simulink model "pointing"  (R2020b)
settings: Solver=ode15s  StartTime=9000  StopTime=15000  MaxStep=1  RelTol=1e-8  AbsTol=1e-8
values from neighbouring files (symbols this model uses):
  data = struct()    [config.m]    (also in config6U.m; configSlew.m; mainOffNominal.m = dataFix; statisticalAnalysis.m = dataFix)
settings Model: SimulationMode=accelerator  Creator=pacif  LastModifiedBy=pacif

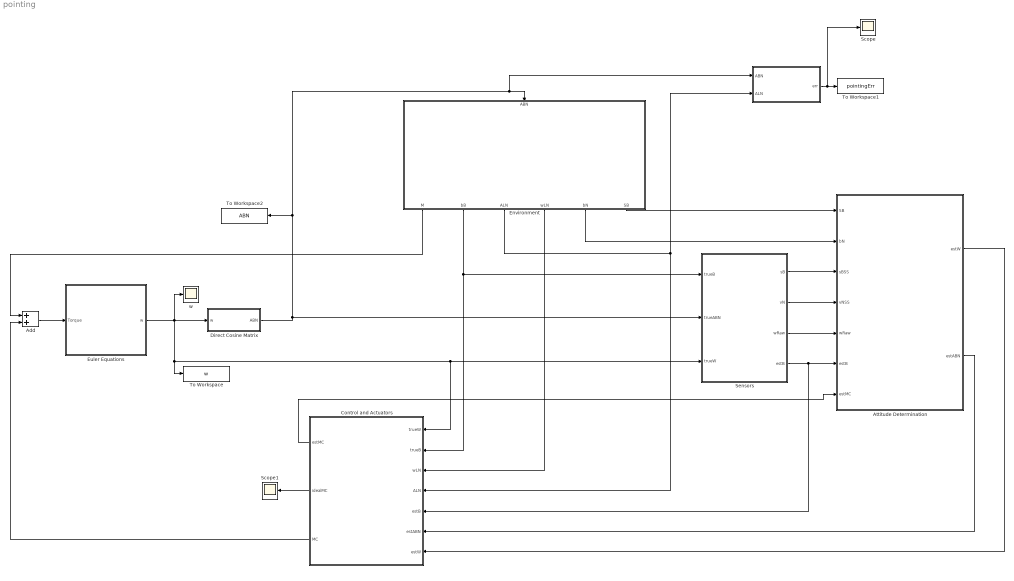
== system pointing ==
  " " : MATLAB Function  TreatAsAtomicUnit=on
  Add : Sum
  Attitude Determination : Subsystem
  Control and Actuators : Subsystem  AncestorBlock=libraryMatlab/Control Logic
  Direct Cosine Matrix : Subsystem  AncestorBlock=libraryMatlab/Direct Cosine Matrix
  Environment : Subsystem  AncestorBlock=libraryMatlab/Environment
  Euler Equations : Subsystem  AncestorBlock=libraryMatlab/Euler Equations
  Scope : Scope
  Scope1 : Scope
  Sensors : Subsystem  AncestorBlock=libraryMatlab/Sensors Old
  To Workspace : ToWorkspace  VariableName=w  SaveFormat=Timeseries  SampleTime=-1
  To Workspace1 : ToWorkspace  VariableName=pointingErr  SaveFormat=Timeseries  SampleTime=-1
  To Workspace2 : ToWorkspace  VariableName=ABN  SaveFormat=Timeseries  SampleTime=-1
  w : Scope
  wires:
  Environment/2(bB) -> Sensors/1(trueB), Control and Actuators/2(trueB)
  Add/1 -> Euler Equations/1(Torque)
  Environment/1(M) -> Add/1
  Euler Equations/1(w) -> Direct Cosine Matrix/1(w), To Workspace/1, Sensors/3(trueW), Control and Actuators/1(trueW), w/1
  Direct Cosine Matrix/1(ABN) -> Sensors/2(trueABN), To Workspace2/1, Environment/1(ABN), " "/1(ABN)
  Environment/3(ALN) -> " "/2(ALN), Control and Actuators/4(ALN)
  Environment/4(wLN) -> Control and Actuators/3(wLN)
  Control and Actuators/3(MC) -> Add/2
  Sensors/1(sB) -> Attitude Determination/3(sBSS)
  Sensors/2(vN) -> Attitude Determination/4(vNSS)
  Sensors/3(wRaw) -> Attitude Determination/5(wRaw)
  Sensors/4(estB) -> Control and Actuators/5(estB), Attitude Determination/6(estB)
  Control and Actuators/1(estMC) -> Attitude Determination/7(estMC)
  Environment/6(SB) -> Attitude Determination/1(SB)
  Environment/5(bN) -> Attitude Determination/2(bN)
  " "/1(err) -> Scope/1, To Workspace1/1
  Attitude Determination/2(estABN) -> Control and Actuators/6(estABN)
  Attitude Determination/1(estW) -> Control and Actuators/7(estW)
  Control and Actuators/2(idealMC) -> Scope1/1

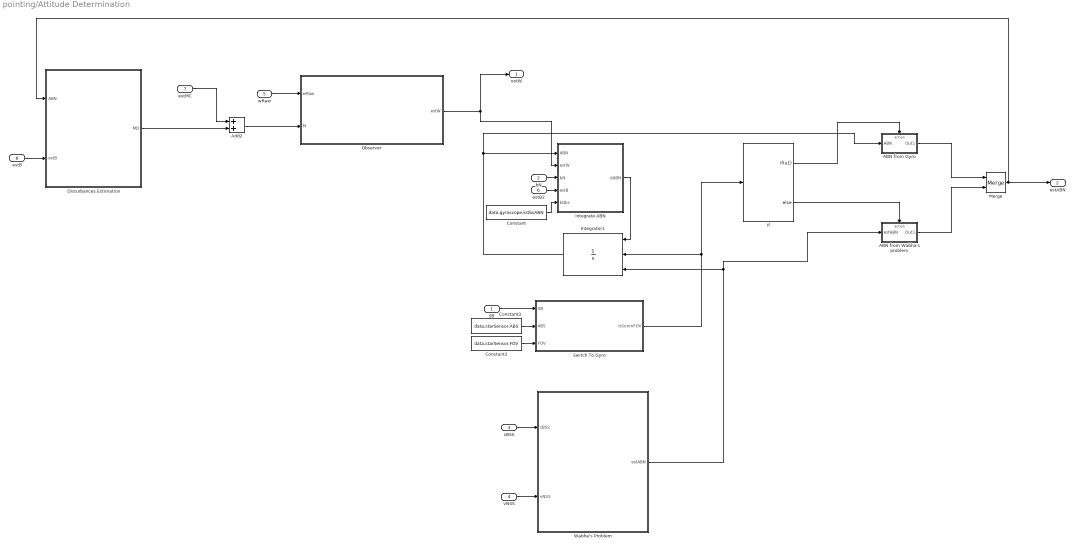
== system pointing/Attitude Determination ==
  SB : Inport
  bN : Inport  Port=2
  sBSS : Inport  Port=3
  vNSS : Inport  Port=4
  wRaw : Inport  Port=5
  estB : Inport  Port=6
  estMC : Inport  Port=7
  ABN from Gyro : Subsystem  TreatAsAtomicUnit=on
  ABN from Wabha's problem : Subsystem  TreatAsAtomicUnit=on
  Add2 : Sum
  Constant : Constant  Value=data.gyroscope.kObsABN
  Constant2 : Constant  Value=data.starSensor.FOV
  Constant3 : Constant  Value=data.starSensor.ABS
  Disturbances Estimation : Subsystem  AncestorBlock=libraryMatlab/Environment
  If : If  IfExpression=u1
  Integrate ABN : MATLAB Function  TreatAsAtomicUnit=on
  Integrator1 : Integrator  ExternalReset=either  InitialConditionSource=external
  Merge : Merge
  Observer : Subsystem
  Switch To Gyro : MATLAB Function  AncestorBlock=libraryMatlab/Is Sun in FOV?  TreatAsAtomicUnit=on
  Wabha's Problem : MATLAB Function  TreatAsAtomicUnit=on
  estB2 : InportShadow  Port=6
  estW : Outport
  estABN : Outport  Port=2
  wires:
  estB/1 -> Disturbances Estimation/2(estB)
  Observer/1(estW) -> estW/1, Integrate ABN/2(estW)
  Add2/1 -> Observer/2(M)
  Disturbances Estimation/1(MD) -> Add2/2
  wRaw/1 -> Observer/1(wRaw)
  estMC/1 -> Add2/1
  Switch To Gyro/1(isSunInFOV) -> If/1, Integrator1/2
  SB/1 -> Switch To Gyro/1(SB)
  Constant2/1 -> Switch To Gyro/3(FOV)
  Constant3/1 -> Switch To Gyro/2(ABS)
  ABN from Wabha's problem/1(Out1) -> Merge/2
  sBSS/1 -> Wabha's Problem/1(sBSS)
  Merge/1 -> Disturbances Estimation/1(ABN), estABN/1
  If/1 -> ABN from Gyro/Action
  Integrator1/1 -> Integrate ABN/1(ABN), ABN from Gyro/1(ABN)
  If/2 -> ABN from Wabha's problem/Action
  Integrate ABN/1(dABN) -> Integrator1/1
  vNSS/1 -> Wabha's Problem/2(vNSS)
  ABN from Gyro/1(Out1) -> Merge/1
  Wabha's Problem/1(estABN) -> ABN from Wabha's problem/1(estABN), Integrator1/3
  bN/1 -> Integrate ABN/3(bN)
  estB2/1 -> Integrate ABN/4(estB)
  Constant/1 -> Integrate ABN/5(kObs)

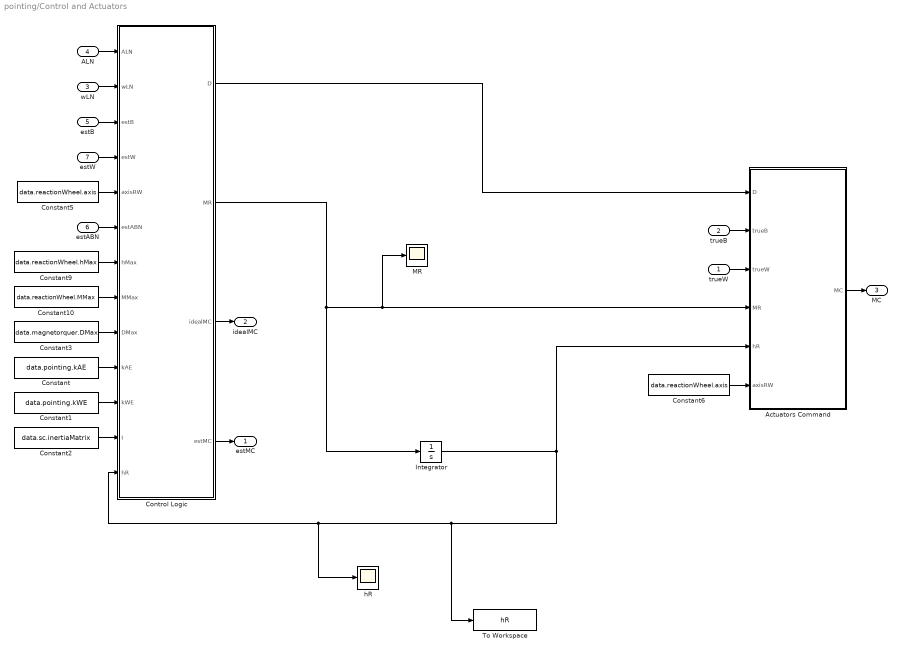
== system pointing/Control and Actuators ==
  trueW : Inport
  trueB : Inport  Port=2
  wLN : Inport  Port=3
  ALN : Inport  Port=4
  estB : Inport  Port=5
  estABN : Inport  Port=6
  estW : Inport  Port=7
  Actuators Command : MATLAB Function  TreatAsAtomicUnit=on
  Constant : Constant  Value=data.pointing.kAE
  Constant1 : Constant  Value=data.pointing.kWE
  Constant10 : Constant  Value=data.reactionWheel.MMax
  Constant2 : Constant  Value=data.sc.inertiaMatrix
  Constant3 : Constant  Value=data.magnetorquer.DMax
  Constant5 : Constant  Value=data.reactionWheel.axis
  Constant6 : Constant  Value=data.reactionWheel.axis
  Constant9 : Constant  Value=data.reactionWheel.hMax
  Control Logic : MATLAB Function  TreatAsAtomicUnit=on
  Integrator : Integrator  InitialCondition=data.reactionWheel.h0
  MR : Scope
  To Workspace : ToWorkspace  VariableName=hR  SaveFormat=Timeseries  SampleTime=-1
  hR : Scope
  estMC : Outport
  idealMC : Outport  Port=2  PortDimensions=3
  MC : Outport  Port=3
  wires:
  estB/1 -> Control Logic/3(estB)
  Constant2/1 -> Control Logic/12(I)
  wLN/1 -> Control Logic/2(wLN)
  estABN/1 -> Control Logic/6(estABN)
  estW/1 -> Control Logic/4(estW)
  Control Logic/3(idealMC) -> idealMC/1
  ALN/1 -> Control Logic/1(ALN)
  Constant5/1 -> Control Logic/5(axisRW)
  Constant3/1 -> Control Logic/9(DMax)
  Actuators Command/1(MC) -> MC/1
  trueB/1 -> Actuators Command/2(trueB)
  Constant6/1 -> Actuators Command/6(axisRW)
  trueW/1 -> Actuators Command/3(trueW)
  Constant9/1 -> Control Logic/7(hMax)
  Constant10/1 -> Control Logic/8(MMax)
  Control Logic/4(estMC) -> estMC/1
  Control Logic/1(D) -> Actuators Command/1(D)
  Control Logic/2(MR) -> Integrator/1, MR/1, Actuators Command/4(MR)
  Integrator/1 -> To Workspace/1, hR/1, Control Logic/13(hR), Actuators Command/5(hR)
  Constant/1 -> Control Logic/10(kAE)
  Constant1/1 -> Control Logic/11(kWE)

== system pointing/Direct Cosine Matrix ==
  w : Inport
  Integrator : Integrator  InitialCondition=data.ic.dcm
  MATLAB Function : MATLAB Function  TreatAsAtomicUnit=on
  MATLAB Function1 : MATLAB Function  TreatAsAtomicUnit=on
  ABN : Outport
  wires:
  MATLAB Function1/1(A) -> MATLAB Function/1(A), ABN/1
  Integrator/1 -> MATLAB Function1/1(A0)
  MATLAB Function/1(dA) -> Integrator/1
  w/1 -> MATLAB Function/2(w)

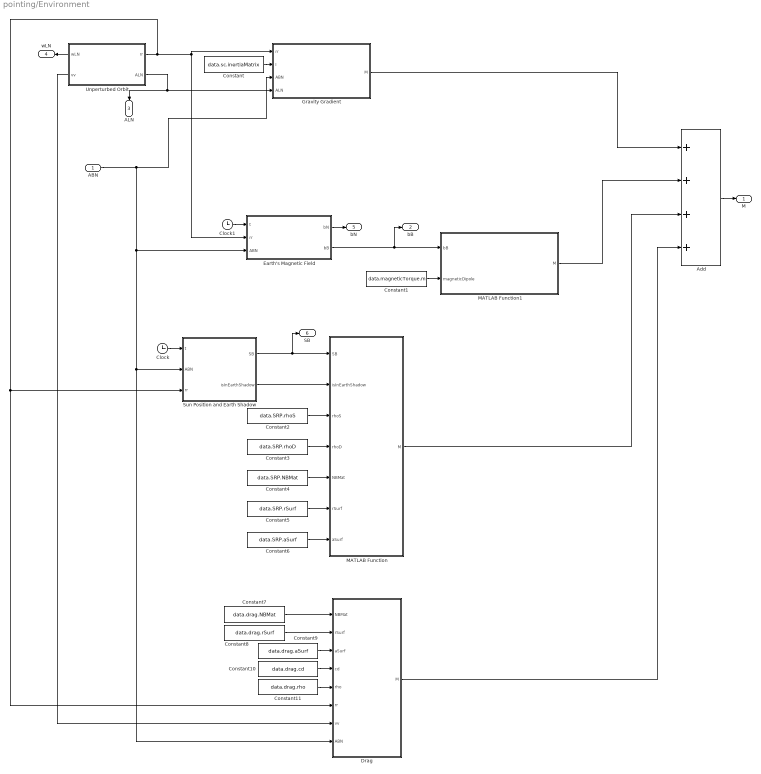
== system pointing/Environment ==
  ABN : Inport
  Add : Sum  Inputs=++++
  Clock : Clock
  Clock1 : Clock
  Constant : Constant  Value=data.sc.inertiaMatrix
  Constant1 : Constant  Value=data.magneticTorque.m
  Constant10 : Constant  Value=data.drag.cd
  Constant11 : Constant  Value=data.drag.rho
  Constant2 : Constant  Value=data.SRP.rhoS
  Constant3 : Constant  Value=data.SRP.rhoD
  Constant4 : Constant  Value=data.SRP.NBMat
  Constant5 : Constant  Value=data.SRP.rSurf
  Constant6 : Constant  Value=data.SRP.aSurf
  Constant7 : Constant  Value=data.drag.NBMat
  Constant8 : Constant  Value=data.drag.rSurf
  Constant9 : Constant  Value=data.drag.aSurf
  Drag : MATLAB Function  TreatAsAtomicUnit=on
  Earth's Magnetic Field : MATLAB Function  TreatAsAtomicUnit=on
  Gravity Gradient : MATLAB Function  TreatAsAtomicUnit=on
  MATLAB Function : MATLAB Function  TreatAsAtomicUnit=on
  MATLAB Function1 : MATLAB Function  TreatAsAtomicUnit=on
  Sun Position and Earth Shadow : MATLAB Function  TreatAsAtomicUnit=on
  Unperturbed Orbit : Subsystem
      settings: PortSchema="{\"entries\":[{\"content\":{\"sides\":[{\"content\":{\"connectorIds\":[\"Out3\",\"Out4\"]},\"type\":\"ConnectorPlacement.EquallySpacedRectSide\",\"uuid\":\"7ed69275-e977-4f2a-8fd3-997b16b83aea\"},{\"content\":{\"connectorIds\":[\"Out1\",\"Out2\"],\"side\":\"RIGHT\"},\"type\":\"ConnectorPlacement.EquallySpacedRectSide\",\"uuid\":\"1b6f9d42-4fef-4598-ba05-7b049053efd9\"},{\"content\":{\"connectorIds\":[],\"side\":\"TOP\"},\"type\":\"ConnectorPlacement.EquallySpacedRectSide\",\"uuid\":\"4e0c3aba-8d31-4992-bec6-35e5e83e5744\"},{\"content\":{\"connectorIds\":[],\"side\":\"HIDDEN\"},\"type\":\"ConnectorPlacement.EquallySpacedRectSide\",\"uuid\":\"810122fe-3bdf-4514-9a6d-d70c18985587\"}]},\"type\":\"ConnectorPlacement.EquallySpacedConnector\",\"uuid\":\"14af5646-8a65-4661-98d5-d8bad349b4d9\"}],\"packageUris\":[\"http://schema.mathworks.com/mf0/Connector/R2020b\"],\"version\":\"1.0\"}"
  M : Outport
  bB : Outport  Port=2
  ALN : Outport  Port=3
  wLN : Outport  Port=4
  bN : Outport  Port=5
  SB : Outport  Port=6
  wires:
  Sun Position and Earth Shadow/1(SB) -> SB/1, MATLAB Function/1(SB)
  Clock/1 -> Sun Position and Earth Shadow/1(t)
  Constant4/1 -> MATLAB Function/5(NBMat)
  Constant6/1 -> MATLAB Function/7(aSurf)
  Constant3/1 -> MATLAB Function/4(rhoD)
  Constant2/1 -> MATLAB Function/3(rhoS)
  Constant5/1 -> MATLAB Function/6(rSurf)
  ABN/1 -> Drag/8(ABN), Sun Position and Earth Shadow/2(ABN), Earth's Magnetic Field/3(ABN), Gravity Gradient/3(ABN)
  Add/1 -> M/1
  MATLAB Function/1(M) -> Add/3
  Gravity Gradient/1(M) -> Add/1
  Earth's Magnetic Field/2(bB) -> MATLAB Function1/1(bB), bB/1
  MATLAB Function1/1(M) -> Add/2
  Constant1/1 -> MATLAB Function1/2(magneticDipole)
  Constant/1 -> Gravity Gradient/2(I)
  Unperturbed Orbit/2(ALN) -> Gravity Gradient/4(ALN), ALN/1
  Unperturbed Orbit/1(rr) -> Sun Position and Earth Shadow/3(rr), Drag/6(rr), Gravity Gradient/1(rr), Earth's Magnetic Field/2(rr)
  Unperturbed Orbit/3(wLN) -> wLN/1
  Clock1/1 -> Earth's Magnetic Field/1(t)
  Constant8/1 -> Drag/2(rSurf)
  Constant9/1 -> Drag/3(aSurf)
  Constant10/1 -> Drag/4(cd)
  Constant7/1 -> Drag/1(NBMat)
  Unperturbed Orbit/4(vv) -> Drag/7(vv)
  Earth's Magnetic Field/1(bN) -> bN/1
  Drag/1(M) -> Add/4
  Constant11/1 -> Drag/5(rho)
  Sun Position and Earth Shadow/2(isInEarthShadow) -> MATLAB Function/2(isInEarthShadow)

== system pointing/Euler Equations ==
  Torque : Inport
  Constant : Constant  Value=data.sc.inertiaMatrix
  Integrator : Integrator  InitialCondition=data.ic.w
  MATLAB Function : MATLAB Function  TreatAsAtomicUnit=on
  w : Outport
  wires:
  MATLAB Function/1(dw) -> Integrator/1
  Torque/1 -> MATLAB Function/2(M)
  Integrator/1 -> MATLAB Function/1(w), w/1
  Constant/1 -> MATLAB Function/3(I)

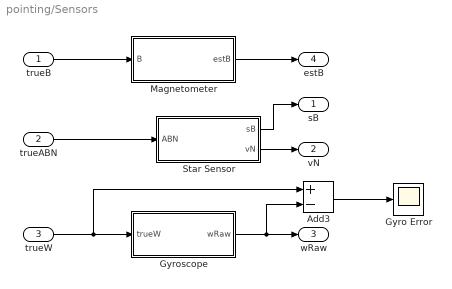
== system pointing/Sensors ==
  trueB : Inport
  trueABN : Inport  Port=2
  trueW : Inport  Port=3
  Add3 : Sum  Inputs=+-
  Gyro Error : Scope
  Gyroscope : Subsystem
  Magnetometer : Subsystem
  Star Sensor : Subsystem  AncestorBlock=libraryMatlab/Sensors/Star Sensor
  sB : Outport
  vN : Outport  Port=2
  wRaw : Outport  Port=3
  estB : Outport  Port=4
  wires:
  Magnetometer/1(estB) -> estB/1
  Add3/1 -> Gyro Error/1
  trueABN/1 -> Star Sensor/1(ABN)
  Star Sensor/1(sB) -> sB/1
  Star Sensor/2(vN) -> vN/1
  Gyroscope/1(wRaw) -> wRaw/1, Add3/2
  trueB/1 -> Magnetometer/1(B)
  trueW/1 -> Add3/1, Gyroscope/1(trueW)

== system pointing/Attitude Determination/ABN from Gyro ==
  ABN : Inport
  Action Port : ActionPort  ActionPortLabel=if(u1)
  Out1 : Outport
  wires:
  ABN/1 -> Out1/1

== system pointing/Attitude Determination/ABN from Wabha's problem ==
  estABN : Inport
  Action Port : ActionPort  ActionPortLabel=else
  Out1 : Outport
  wires:
  estABN/1 -> Out1/1

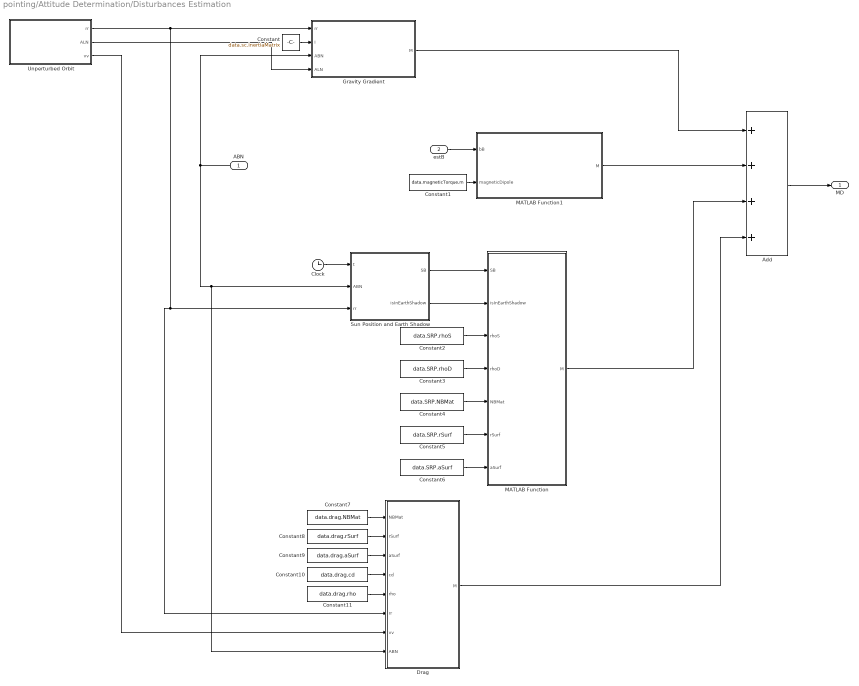
== system pointing/Attitude Determination/Disturbances Estimation ==
  ABN : Inport
  estB : Inport  Port=2
  Add : Sum  Inputs=++++
  Clock : Clock
  Constant : Constant  Value=data.sc.inertiaMatrix
  Constant1 : Constant  Value=data.magneticTorque.m
  Constant10 : Constant  Value=data.drag.cd
  Constant11 : Constant  Value=data.drag.rho
  Constant2 : Constant  Value=data.SRP.rhoS
  Constant3 : Constant  Value=data.SRP.rhoD
  Constant4 : Constant  Value=data.SRP.NBMat
  Constant5 : Constant  Value=data.SRP.rSurf
  Constant6 : Constant  Value=data.SRP.aSurf
  Constant7 : Constant  Value=data.drag.NBMat
  Constant8 : Constant  Value=data.drag.rSurf
  Constant9 : Constant  Value=data.drag.aSurf
  Drag : MATLAB Function  TreatAsAtomicUnit=on
  Gravity Gradient : MATLAB Function  TreatAsAtomicUnit=on
  MATLAB Function : MATLAB Function  TreatAsAtomicUnit=on
  MATLAB Function1 : MATLAB Function  TreatAsAtomicUnit=on
  Sun Position and Earth Shadow : MATLAB Function  TreatAsAtomicUnit=on
  Unperturbed Orbit : Subsystem
  MD : Outport
  wires:
  Constant7/1 -> Drag/1(NBMat)
  Constant6/1 -> MATLAB Function/7(aSurf)
  ABN/1 -> Sun Position and Earth Shadow/2(ABN), Drag/8(ABN), Gravity Gradient/3(ABN)
  Constant2/1 -> MATLAB Function/3(rhoS)
  Drag/1(M) -> Add/4
  Constant4/1 -> MATLAB Function/5(NBMat)
  Sun Position and Earth Shadow/1(SB) -> MATLAB Function/1(SB)
  Sun Position and Earth Shadow/2(isInEarthShadow) -> MATLAB Function/2(isInEarthShadow)
  Constant/1 -> Gravity Gradient/2(I)
  Constant1/1 -> MATLAB Function1/2(magneticDipole)
  Gravity Gradient/1(M) -> Add/1
  Constant8/1 -> Drag/2(rSurf)
  Clock/1 -> Sun Position and Earth Shadow/1(t)
  Constant3/1 -> MATLAB Function/4(rhoD)
  MATLAB Function1/1(M) -> Add/2
  Unperturbed Orbit/1(rr) -> Gravity Gradient/1(rr), Drag/6(rr), Sun Position and Earth Shadow/3(rr)
  Constant9/1 -> Drag/3(aSurf)
  Unperturbed Orbit/2(ALN) -> Gravity Gradient/4(ALN)
  Unperturbed Orbit/3(vv) -> Drag/7(vv)
  Constant10/1 -> Drag/4(cd)
  Add/1 -> MD/1
  MATLAB Function/1(M) -> Add/3
  Constant11/1 -> Drag/5(rho)
  Constant5/1 -> MATLAB Function/6(rSurf)
  estB/1 -> MATLAB Function1/1(bB)

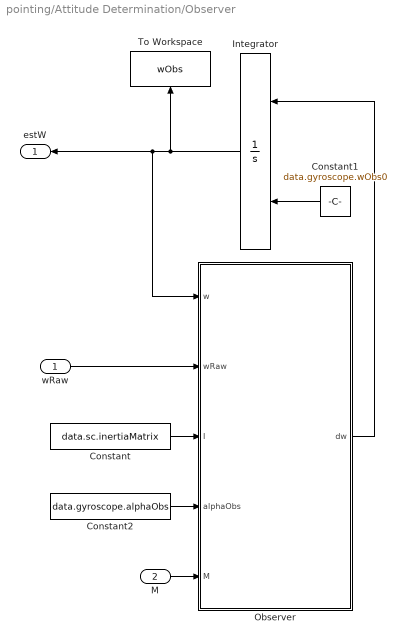
== system pointing/Attitude Determination/Observer ==
  wRaw : Inport
  M : Inport  Port=2
  Constant : Constant  Value=data.sc.inertiaMatrix
  Constant1 : Constant  Value=data.gyroscope.wObs0
  Constant2 : Constant  Value=data.gyroscope.alphaObs
  Integrator : Integrator  InitialConditionSource=external
  Observer : MATLAB Function  TreatAsAtomicUnit=on
  To Workspace : ToWorkspace  VariableName=wObs  SaveFormat=Timeseries  SampleTime=-1
  estW : Outport
  wires:
  Constant1/1 -> Integrator/2
  M/1 -> Observer/5(M)
  Constant2/1 -> Observer/4(alphaObs)
  Integrator/1 -> To Workspace/1, Observer/1(w), estW/1
  Observer/1(dw) -> Integrator/1
  Constant/1 -> Observer/3(I)
  wRaw/1 -> Observer/2(wRaw)

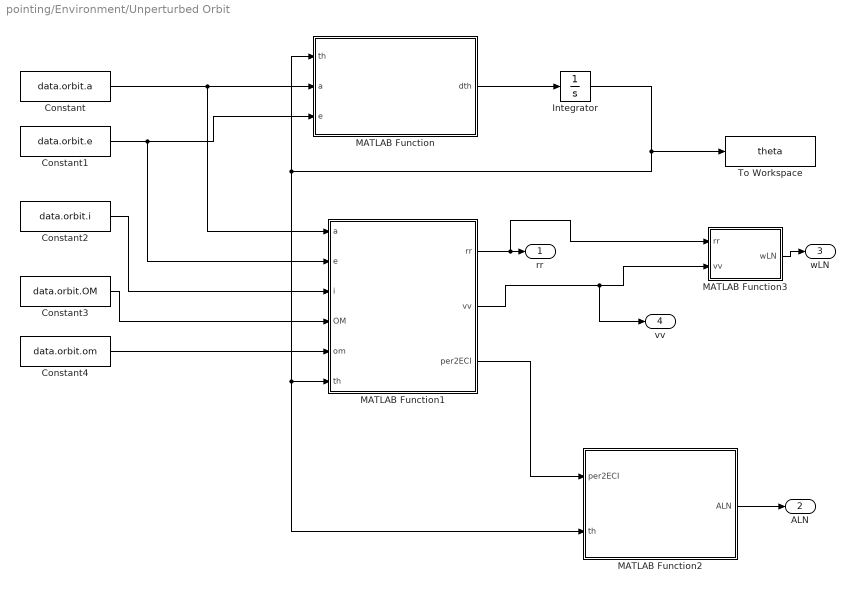
== system pointing/Environment/Unperturbed Orbit ==
  Constant : Constant  Value=data.orbit.a
  Constant1 : Constant  Value=data.orbit.e
  Constant2 : Constant  Value=data.orbit.i
  Constant3 : Constant  Value=data.orbit.OM
  Constant4 : Constant  Value=data.orbit.om
  Integrator : Integrator  InitialCondition=data.ic.th
  MATLAB Function : MATLAB Function  TreatAsAtomicUnit=on
  MATLAB Function1 : MATLAB Function  TreatAsAtomicUnit=on
  MATLAB Function2 : MATLAB Function  TreatAsAtomicUnit=on
  MATLAB Function3 : MATLAB Function  TreatAsAtomicUnit=on
  To Workspace : ToWorkspace  VariableName=theta  SaveFormat=Timeseries  SampleTime=-1
  rr : Outport
  ALN : Outport  Port=2
  wLN : Outport  Port=3
  vv : Outport  Port=4
  wires:
  MATLAB Function3/1(wLN) -> wLN/1
  MATLAB Function2/1(ALN) -> ALN/1
  MATLAB Function1/3(per2ECI) -> MATLAB Function2/1(per2ECI)
  MATLAB Function1/2(vv) -> vv/1, MATLAB Function3/2(vv)
  MATLAB Function1/1(rr) -> rr/1, MATLAB Function3/1(rr)
  Constant4/1 -> MATLAB Function1/5(om)
  Constant3/1 -> MATLAB Function1/4(OM)
  Constant2/1 -> MATLAB Function1/3(i)
  Integrator/1 -> MATLAB Function/1(th), MATLAB Function1/6(th), MATLAB Function2/2(th), To Workspace/1
  MATLAB Function/1(dth) -> Integrator/1
  Constant1/1 -> MATLAB Function/3(e), MATLAB Function1/2(e)
  Constant/1 -> MATLAB Function/2(a), MATLAB Function1/1(a)

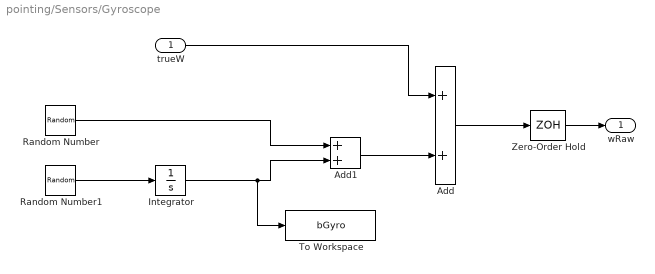
== system pointing/Sensors/Gyroscope ==
  trueW : Inport
  Add : Sum
  Add1 : Sum
  Integrator : Integrator  InitialCondition=data.gyroscope.b0
  Random Number : RandomNumber  Variance=data.gyroscope.sigmaN^2*[1;1;1]  Seed=[2323; 3445;34]  SampleTime=data.gyroscope.sampleTime
  Random Number1 : RandomNumber  Variance=data.gyroscope.sigmaB^2*[1;1;1]  Seed=[34432; 345456;1087]  SampleTime=data.gyroscope.sampleTime
  To Workspace : ToWorkspace  VariableName=bGyro  SaveFormat=Timeseries  SampleTime=-1
  Zero-Order Hold : ZeroOrderHold  SampleTime=data.gyroscope.sampleTime
  wRaw : Outport
  wires:
  Zero-Order Hold/1 -> wRaw/1
  Add/1 -> Zero-Order Hold/1
  Random Number/1 -> Add1/1
  Add1/1 -> Add/2
  trueW/1 -> Add/1
  Integrator/1 -> To Workspace/1, Add1/2
  Random Number1/1 -> Integrator/1

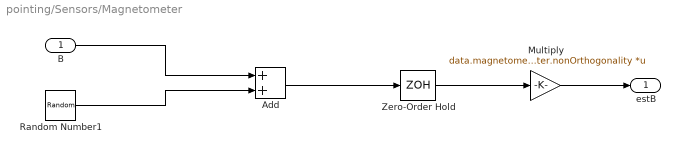
== system pointing/Sensors/Magnetometer ==
  B : Inport
  Add : Sum
  Multiply : Gain  Gain=data.magnetometer.nonOrthogonality  Multiplication=Matrix(K*u) (u vector)
  Random Number1 : RandomNumber  Variance=(data.magnetometer.sigma)^2*[1;1;1]  Seed=randi(1e5,3,1)  SampleTime=data.magnetometer.sampleTime
  Zero-Order Hold : ZeroOrderHold  SampleTime=data.magnetometer.sampleTime
  estB : Outport
  wires:
  Random Number1/1 -> Add/2
  Add/1 -> Zero-Order Hold/1
  B/1 -> Add/1
  Zero-Order Hold/1 -> Multiply/1
  Multiply/1 -> estB/1

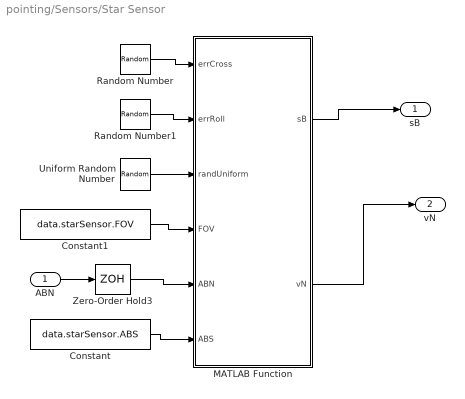
== system pointing/Sensors/Star Sensor ==
  ABN : Inport
  Constant : Constant  Value=data.starSensor.ABS
  Constant1 : Constant  Value=data.starSensor.FOV
  MATLAB Function : MATLAB Function  TreatAsAtomicUnit=on
  Random Number : RandomNumber  Variance=data.starSensor.sigmaCross^2*ones(2*data.starSensor.NStars,1)  Seed=randi(1e5,2*data.starSensor.NStars,1)  SampleTime=data.starSensor.sampleTime  VectorParams1D=off
  Random Number1 : RandomNumber  Variance=data.starSensor.sigmaRoll^2*ones(data.starSensor.NStars,1)  Seed=randi(1e5,data.starSensor.NStars,1)  SampleTime=data.starSensor.sampleTime
  Uniform Random Number : UniformRandomNumber  Seed=randi(1e5,data.starSensor.NStars*2,1)  SampleTime=data.starSensor.sampleTime
  Zero-Order Hold3 : ZeroOrderHold  SampleTime=data.starSensor.sampleTime
  sB : Outport
  vN : Outport  Port=2
  wires:
  Constant/1 -> MATLAB Function/6(ABS)
  Constant1/1 -> MATLAB Function/4(FOV)
  ABN/1 -> Zero-Order Hold3/1
  MATLAB Function/1(sB) -> sB/1
  MATLAB Function/2(vN) -> vN/1
  Random Number/1 -> MATLAB Function/1(errCross)
  Zero-Order Hold3/1 -> MATLAB Function/5(ABN)
  Random Number1/1 -> MATLAB Function/2(errRoll)
  Uniform Random Number/1 -> MATLAB Function/3(randUniform)

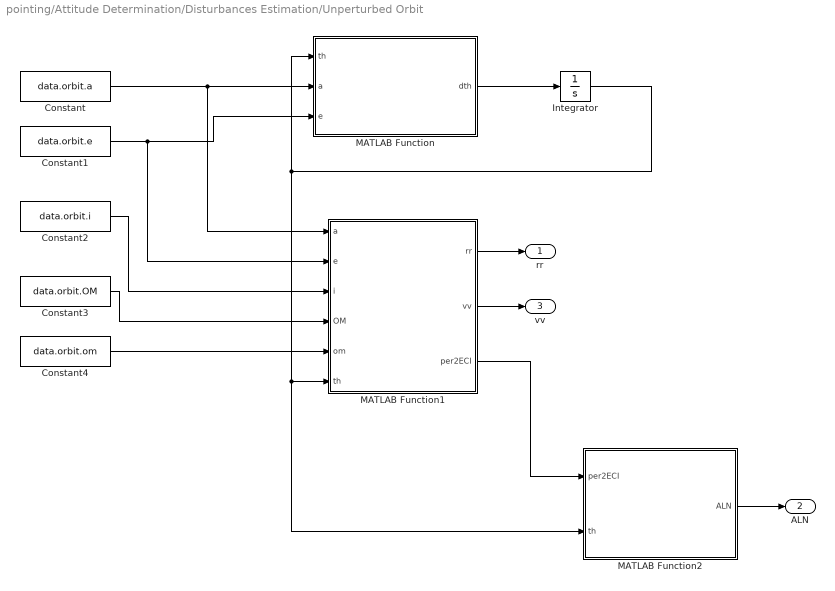
== system pointing/Attitude Determination/Disturbances Estimation/Unperturbed Orbit ==
  Constant : Constant  Value=data.orbit.a
  Constant1 : Constant  Value=data.orbit.e
  Constant2 : Constant  Value=data.orbit.i
  Constant3 : Constant  Value=data.orbit.OM
  Constant4 : Constant  Value=data.orbit.om
  Integrator : Integrator  InitialCondition=data.ic.th
  MATLAB Function : MATLAB Function  TreatAsAtomicUnit=on
  MATLAB Function1 : MATLAB Function  TreatAsAtomicUnit=on
  MATLAB Function2 : MATLAB Function  TreatAsAtomicUnit=on
  rr : Outport
  ALN : Outport  Port=2
  vv : Outport  Port=3
  wires:
  MATLAB Function2/1(ALN) -> ALN/1
  MATLAB Function1/3(per2ECI) -> MATLAB Function2/1(per2ECI)
  MATLAB Function1/2(vv) -> vv/1
  MATLAB Function1/1(rr) -> rr/1
  Constant4/1 -> MATLAB Function1/5(om)
  Constant3/1 -> MATLAB Function1/4(OM)
  Constant2/1 -> MATLAB Function1/3(i)
  Integrator/1 -> MATLAB Function/1(th), MATLAB Function1/6(th), MATLAB Function2/2(th)
  MATLAB Function/1(dth) -> Integrator/1
  Constant1/1 -> MATLAB Function/3(e), MATLAB Function1/2(e)
  Constant/1 -> MATLAB Function/2(a), MATLAB Function1/1(a)

== matlab function pointing/Environment/Unperturbed Orbit/MATLAB Function1 ==
  data: a input; rr output; e input; i input; OM input; om input; th input; vv output; per2ECI output
function [rr,vv,per2ECI] = kep2car(a,e,i,OM,om,th)

MU = 398600;

p = a*(1-e^2);
r = p/(1+e*cos(th));

rr = r*[cos(th);sin(th);0];
vv = sqrt(MU/p)*[-sin(th);e+cos(th);0];

ROM = [ cos(OM) sin(OM) 0; -sin(OM) cos(OM) 0; 0 0 1];
Ri = [ 1 0 0; 0 cos(i) sin(i); 0 -sin(i) cos(i)];
Rom = [ cos(om) sin(om) 0; -sin(om) cos(om) 0; 0 0 1];

per2ECI = (Rom*Ri*ROM)';

rr = per2ECI*rr;
vv = per2ECI*vv;

end

== matlab function pointing/Environment/Unperturbed Orbit/MATLAB Function2 ==
  data: per2ECI input; ALN output; th input
function ALN = computeALN(per2ECI,th)

ECI2per = per2ECI';

per2L = [cos(th)  sin(th)  0;
        -sin(th)  cos(th)  0;
            0        0     1];
        
ALN = per2L*ECI2per;

end

== matlab function pointing/Environment/MATLAB Function1 ==
  data: bB input; M output; magneticDipole input
function M = magneticTorque(bB,magneticDipole)

M = cross(magneticDipole,bB); 

end

== matlab function pointing/Environment/MATLAB Function ==
  data: SB input; isInEarthShadow input; rhoS input; rhoD input; NBMat input; rSurf input; aSurf input; M output
function M = SRP(SB,isInEarthShadow,rhoS,rhoD,NBMat,rSurf,aSurf)

% Constants:
Fe = 2081.4; c = 3e8; P = Fe/c;

nSurf = size(NBMat,2);

M = [0; 0; 0];

if ~isInEarthShadow
    
    for i = 1:nSurf
        
        NBi = NBMat(:,i); ri = rSurf(:,i); Ai = aSurf(i);
        rhoSi = rhoS(i); rhoDi = rhoD(i);
        
        Ki = dot(SB,NBi);
        
        if Ki > 0
            
            Fi = -P*Ai*Ki*((1-rhoSi)*SB +...
                (2*rhoSi*Ki + 2/3*rhoDi)*NBi);
            
            M = M + cross(ri,Fi);
            
        end
        
    end
    
end
end

== matlab function pointing/Environment/Drag ==
  data: NBMat input; M output; rSurf input; aSurf input; cd input; rho input; rr input; vv input; ABN input
function M = fcn(NBMat,rSurf,aSurf,cd,rho,rr,vv,ABN)

wEarth = 0.000072921;

rr = rr*1e3; vv = vv*1e3;

vRel = ABN*[vv(1) + wEarth*rr(1); vv(2) - wEarth*rr(2); vv(3)];

nSurf = size(NBMat,2);

M = [0; 0; 0];

for i = 1:nSurf
    
    NBi = NBMat(:,i); ri = rSurf(:,i); Ai = aSurf(i);
    
    Ki = dot(vRel/norm(vRel),NBi); 
    
    if Ki > 0
        
        Fi = -0.5*rho*cd*norm(vRel)*vRel*Ai*Ki;
        
        M = M + cross(ri,Fi);
        
    end
    
end

end

== matlab function pointing/Attitude Determination/Disturbances Estimation/Drag ==
  data: NBMat input; M output; rSurf input; aSurf input; cd input; rho input; rr input; vv input; ABN input
function M = fcn(NBMat,rSurf,aSurf,cd,rho,rr,vv,ABN)

wEarth = 0.000072921;

rr = rr*1e3; vv = vv*1e3;

vRel = ABN*[vv(1) + wEarth*rr(1); vv(2) - wEarth*rr(2); vv(3)];

nSurf = size(NBMat,2);

M = [0; 0; 0];

for i = 1:nSurf
    
    NBi = NBMat(:,i); ri = rSurf(:,i); Ai = aSurf(i);
    
    Ki = dot(vRel/norm(vRel),NBi); 
    
    if Ki > 0
        
        Fi = -0.5*rho*cd*norm(vRel)*vRel*Ai*Ki;
        
        M = M + cross(ri,Fi);
        
    end
    
end

end

== matlab function pointing/Control and Actuators/Actuators Command ==
  data: D input; MC output; trueB input; trueW input; MR input; hR input; axisRW input
function MC  = fcn(D, trueB, trueW, MR, hR, axisRW)

MC = [0;0;0];

% Magnetorquers:
MMagn = cross(D,trueB);

% Reaction Wheels:
MRW = -cross(trueW,axisRW*hR) - axisRW*MR;

MC = MMagn + MRW;

== matlab function pointing/Attitude Determination/Disturbances Estimation/Gravity Gradient ==
  data: rr input; M output; I input; ABN input; ALN input
function M = fun(rr,I,ABN,ALN)

MU = 398600;

Ix = I(1,1); Iy = I(2,2); Iz = I(3,3);

R = norm(rr);

ABL = ABN*ALN';

c = ABL*[1;0;0];

K = 3*MU/R^3;

M = K*[ (Iz - Iy)*c(3)*c(2);
        (Ix - Iz)*c(1)*c(3);
        (Iy - Ix)*c(2)*c(1)  ];
    
end

== matlab function pointing/Attitude Determination/Disturbances Estimation/MATLAB Function ==
  data: SB input; isInEarthShadow input; rhoS input; rhoD input; NBMat input; rSurf input; aSurf input; M output
function M = SRP(SB,isInEarthShadow,rhoS,rhoD,NBMat,rSurf,aSurf)

% Constants:
Fe = 2081.4; c = 3e8; P = Fe/c;

nSurf = size(NBMat,2);

M = [0; 0; 0];

if ~isInEarthShadow
    
    for i = 1:nSurf
        
        NBi = NBMat(:,i); ri = rSurf(:,i); Ai = aSurf(i);
        rhoSi = rhoS(i); rhoDi = rhoD(i);
        
        Ki = dot(SB,NBi);
        
        if Ki > 0
            
            Fi = -P*Ai*Ki*((1-rhoSi)*SB +...
                (2*rhoSi*Ki + 2/3*rhoDi)*NBi);
            
            M = M + cross(ri,Fi);
            
        end
        
    end
    
end
end

== matlab function pointing/Attitude Determination/Disturbances Estimation/MATLAB Function1 ==
  data: bB input; M output; magneticDipole input
function M = magneticTorque(bB,magneticDipole)

M = cross(magneticDipole,bB); 

end

== matlab function pointing/Attitude Determination/Disturbances Estimation/Sun Position and Earth Shadow ==
  data: t input; SB output; ABN input; rr input; isInEarthShadow output
function [SB,isInEarthShadow] = fcn(t,ABN,rr)

N_SUN = 2*pi/365/24/3600; OBL = 23.45*pi/180;
R_SUN = 1.496e8; R_EARTH = 6378;

rSun = R_SUN*[cos(N_SUN*t); 
    sin(N_SUN*t)*cos(OBL);
    sin(N_SUN*t)*sin(OBL)];

SB = ABN*rSun/norm(rSun);

% Check if satellite is in Earth's shadow:

th = acos(dot(rSun,rr)/norm(rSun)/norm(rr));
th1 = acos(R_EARTH/norm(rr)); 
th2 = acos(R_EARTH/norm(rSun)); 

isInEarthShadow = th > th1 + th2;

== matlab function pointing/Environment/Earth's Magnetic Field ==
  data: bN output; t input; bB output; rr input; ABN input
function [bN,bB] = fcn(t,rr,ABN)

% Coefficients for 2020:
g10 = -29615e-9; g11 = -1728e-9; h11 = 5186e-9;
H0 = sqrt(g10^2 + g11^2 + h11^2);

OBL = 11.5*pi/180;
W_EARTH = (2*pi + 2*pi/365.26)/24/3600;
R_EARTH = 6371.0088;

mVers = [sin(OBL)*cos(W_EARTH*t);
        sin(OBL)*sin(W_EARTH*t);
        cos(OBL)];

rVers = rr/norm(rr);
rNorm = norm(rr);

bN = R_EARTH^3/rNorm^3*H0*(3*dot(mVers,rVers)*rVers - mVers);

bB = ABN*bN;

end

== matlab function pointing/Attitude Determination/Disturbances Estimation/Unperturbed Orbit/MATLAB Function ==
  data: th input; dth output; a input; e input
function dth = thetaDot(th, a, e)

MU = 398600;

n = sqrt(MU/a^3);

dth = n*(1 + e*cos(th))^2/(1 - e^2)^(3/2);

end

== matlab function pointing/Attitude Determination/Disturbances Estimation/Unperturbed Orbit/MATLAB Function1 ==
  data: a input; rr output; e input; i input; OM input; om input; th input; vv output; per2ECI output
function [rr,vv,per2ECI] = kep2car(a,e,i,OM,om,th)

MU = 398600;

p = a*(1-e^2);
r = p/(1+e*cos(th));

rr = r*[cos(th);sin(th);0];
vv = sqrt(MU/p)*[-sin(th);e+cos(th);0];

ROM = [ cos(OM) sin(OM) 0; -sin(OM) cos(OM) 0; 0 0 1];
Ri = [ 1 0 0; 0 cos(i) sin(i); 0 -sin(i) cos(i)];
Rom = [ cos(om) sin(om) 0; -sin(om) cos(om) 0; 0 0 1];

per2ECI = (Rom*Ri*ROM)';

rr = per2ECI*rr;
vv = per2ECI*vv;

end

== matlab function pointing/Attitude Determination/Disturbances Estimation/Unperturbed Orbit/MATLAB Function2 ==
  data: per2ECI input; ALN output; th input
function ALN = computeALN(per2ECI,th)

ECI2per = per2ECI';

per2L = [cos(th)  sin(th)  0;
        -sin(th)  cos(th)  0;
            0        0     1];
        
ALN = per2L*ECI2per;

end

== matlab function pointing/Environment/Unperturbed Orbit/MATLAB Function3 ==
  data: rr input; wLN output; vv input
function wLN = fcn(rr,vv)

MU = 398600;

n = sqrt(MU/(norm(rr)^3));

h = cross(rr,vv); 

wLN = h/norm(h)*n;

== matlab function pointing/Environment/Sun Position and Earth Shadow ==
  data: t input; SB output; ABN input; rr input; isInEarthShadow output
function [SB,isInEarthShadow] = fcn(t,ABN,rr)

N_SUN = 2*pi/365/24/3600; OBL = 23.45*pi/180;
R_SUN = 1.496e8; R_EARTH = 6378;

rSun = R_SUN*[cos(N_SUN*t); 
    sin(N_SUN*t)*cos(OBL);
    sin(N_SUN*t)*sin(OBL)];

SB = ABN*rSun/norm(rSun);

% Check if satellite is in Earth's shadow:

th = acos(dot(rSun,rr)/norm(rSun)/norm(rr));
th1 = acos(R_EARTH/norm(rr)); 
th2 = acos(R_EARTH/norm(rSun)); 

isInEarthShadow = th > th1 + th2;

== matlab function pointing/Sensors/Star Sensor/MATLAB Function ==
  data: errCross input; errRoll input; randUniform input; sB output; FOV input; ABN input; ABS input; vN output
function [sB,vN] = fcn(errCross,errRoll,randUniform,FOV,ABN,ABS)

N = length(errRoll);

A_NS = ABN'*ABS;

sB = zeros(3,N); vN = sB;

for i = 1:N
    
    a = randUniform(2*i-1)*FOV/2; b = randUniform(2*i)*pi/2;
    
    vS = [sin(b)*cos(a); sin(b)*sin(a); cos(b)];
    
    phi = errCross(2*i-1); theta = errCross(2*i); psi = errRoll(i);
    
    errA123 = [ cos(psi)*cos(theta), cos(phi)*sin(psi) + cos(psi)*sin(phi)*sin(theta), sin(phi)*sin(psi) - cos(phi)*cos(psi)*sin(theta)
                -cos(theta)*sin(psi), cos(phi)*cos(psi) - sin(phi)*sin(psi)*sin(theta), cos(psi)*sin(phi) + cos(phi)*sin(psi)*sin(theta)
                sin(theta),                             -cos(theta)*sin(phi),                              cos(phi)*cos(theta)];
    sS = errA123*vS;
    
    sB(:,i) = ABS*sS; vN(:,i) = A_NS*vS;
end

== matlab function pointing/Control and Actuators/Control Logic ==
  data: ALN input; wLN input; estB input; estW input; axisRW input; D output; MR output; idealMC output; estABN input; estMC output; hMax input; MMax input; DMax input; kAE input; kWE input; I input; hR input
function [D,MR,idealMC,estMC] = fcn(ALN,wLN,estB,estW,axisRW,estABN,...
                                    hMax,MMax,DMax,kAE,kWE,I,hR)

D = [0;0;0]; MR = 0; idealMC = [0;0;0]; estMC = [0;0;0];

AD = ALN;

wD = ALN*wLN;

AE = estABN*AD';

wE = estW - AE*wD;

AEV = [AE(2,3) - AE(3,2);
    AE(3,1) - AE(1,3);
    AE(1,2) - AE(2,1)];

idealMC = -kWE*wE - kAE*AEV + cross(estW,I*estW) -...
    I*cross(wE,AE*wD);

MC1 = idealMC + cross(estW,axisRW*hR);

D = cross(estB,MC1)/norm(estB)^2;

% Check on values of D:
D = max(D,-DMax); D = min(D,DMax);

MC2 = MC1 - cross(D,estB);

MR = -dot(MC2,axisRW);

% Checks on MR:
if abs(hR) > hMax && MR*hR>0, MR = 0; end
if abs(MR) > MMax, MR = sign(MR)*MMax; end

estMC = cross(D,estB) - MR*axisRW - cross(estW,hR*axisRW);

== matlab function pointing/Attitude Determination/Observer/Observer ==
  data: w input; dw output; wRaw input; I input; alphaObs input; M input
function dw = fcn(w,wRaw,I,alphaObs,M)

dw = I\cross(I*w,w) + I\M - alphaObs*(w - wRaw);

== matlab function pointing/Attitude Determination/Switch To Gyro ==
  data: SB input; isSunInFOV output; ABS input; FOV input
function isSunInFOV = fcn(SB,ABS,FOV)

% Sun in FOV:
SS = ABS'*SB;

alphaS = acos(SS(3));

isSunInFOV = alphaS < FOV/2;

== matlab function pointing/Attitude Determination/Wabha's Problem ==
  data: estABN output; sBSS input; vNSS input
function estABN  = fcn(sBSS,vNSS)

estABN = zeros(3);

nS = size(sBSS,2);

B = zeros(3);

for iS = 1:nS
    
    B = B + 1/nS*sBSS(:,iS)*vNSS(:,iS)';
    
end

[U,~,V] = svd(B);

M = diag([1,1,det(U)*det(V)]);
estABN = real(U*M*V');

== matlab function pointing/Direct Cosine Matrix/MATLAB Function ==
  data: A input; dA output; w input
function dA = derivativeDCM(A,w)

M = [ 0 -w(3) w(2); 
    w(3) 0 -w(1);
    -w(2) w(1) 0];

dA = -M*A;


end

== matlab function pointing/Euler Equations/MATLAB Function ==
  data: w input; dw output; M input; I input
function dw = eulerEquations(w,M,I)

dw = I\(cross(I*w,w) + M);

end

== matlab function pointing/Direct Cosine Matrix/MATLAB Function1 ==
  data: A0 input; A output
function A = orthonormalizeA(A0)

A = A0*3/2 - A0*(A0')*A0/2;

end

== matlab function pointing/  ==
  data: ABN input; err output; ALN input
function err = fcn(ABN,ALN)

ABL = ABN*ALN';

err = acosd(diag(ABL));

== matlab function pointing/Attitude Determination/Integrate ABN ==
  data: ABN input; dABN output; estW input; bN input; estB input; kObs input
function dABN = fcn(ABN,estW,bN,estB,kObs)

alpha = kObs*cross(estB,ABN*bN)/norm(estB)/norm(bN);

wPlusAlpha = alpha + estW;

W = [0 -wPlusAlpha(3) wPlusAlpha(2); wPlusAlpha(3) 0 -wPlusAlpha(1); -wPlusAlpha(2) wPlusAlpha(1) 0];

dABN = -W*ABN;

== matlab function pointing/Environment/Gravity Gradient ==
  data: rr input; M output; I input; ABN input; ALN input
function M = fun(rr,I,ABN,ALN)

MU = 398600;

Ix = I(1,1); Iy = I(2,2); Iz = I(3,3);

R = norm(rr);

ABL = ABN*ALN';

c = ABL*[1;0;0];

K = 3*MU/R^3;

M = K*[ (Iz - Iy)*c(3)*c(2);
        (Ix - Iz)*c(1)*c(3);
        (Iy - Ix)*c(2)*c(1)  ];
    
end

== matlab function pointing/Environment/Unperturbed Orbit/MATLAB Function ==
  data: th input; dth output; a input; e input
function dth = thetaDot(th, a, e)

MU = 398600;

n = sqrt(MU/a^3);

dth = n*(1 + e*cos(th))^2/(1 - e^2)^(3/2);

end
